simulink library "powerlib"  (Simulink 6.0)
settings: Solver=ode45  SolverMode=SingleTasking  StartTime=0.0  StopTime=10.0  RelTol=1e-3
undefined symbols (not defined in the file or in its folder): com, ctrl1, Da, DiscIntNeverNeededParam, dtha, etat, FA, find_system, Ha, j, Ka, Ki, Kv, q0, Rground, sel, st_a, st_b, st_c, sta, stb, stc, T1, T2, T3, T4
libraries: powerlib_models x30, powerlib x25, simulink_extras x6, powerlib_extras x3, simulink x2
(part 2 of 7)

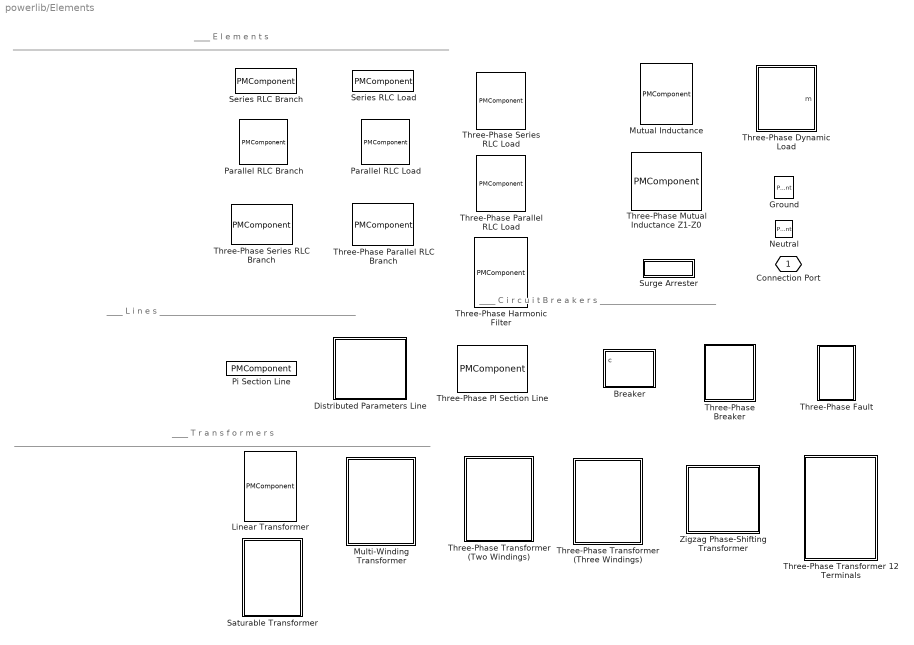
== system powerlib/Elements ==
  note: ____ T r a n s f o r m e r s ________________________________________________________________________________________________________
  note: ____ C i r c u i t B r e a k e r s _____________________________
  note: ____ L i n e s _________________________________________________
  note: ____ E l e m e n t s _____________________________________________________________________________________________________________
  Breaker : Subsystem  mask(Breaker){BreakerResistance=0.01, InitialState=0, SnubberResistance=1e6, SnubberCapacitance=inf, SwitchingTimes=[ 1/60  5/60 ], External=on, Measurements=None}
      mask prompts: BreakerResistance "Breaker resistance Ron (Ohm):"; InitialState "Initial state ( 0 for 'open' , 1 for 'closed' ):"; SnubberResistance "Snubber resistance Rs (Ohms):"; SnubberCapacitance "Snubber capacitance Cs (F):"; SwitchingTimes "Switching times (s):"; External "External control of switching times"
      mask help:
      | Implements a circuit breaker with internal resistance Ron. Ron is required by the
      | model  and cannot be set to zero.
      |
      | When the external control mode is selected, a Simulink  logical signal is used to
      | control the breaker operation.  When  the signal becomes greater than zero the
      | breaker closes instantaneously.  When it becomes zero, the breaker opens at the
      | next current zero-crossing.
      mask init:
      | block = gcb;
      | [p0,p1,p3,s1,s2,com,switchings]=powericon('Breaker',InitialState,SnubberResistance,SnubberCapacitance,SwitchingTimes,External);
      | powericon('BreakerCback',block);
      | powericon('psbloadfunction',block,'goto','Initialize');
      settings: CopyFcn=powericon('psbloadfunction',gcb,'goto','UpdateGotoTag');
      mask Help: web(psbhelp);
      mask StyleString: edit,edit,edit,edit,edit,checkbox,popup(None|Branch voltage|Branch current|Branch voltage and current)
      mask CallbackString: |||||powericon('BreakerCback',gcb);|
      mask Display: plot(p0,25,p1,75,[15,15,25,25,15],[55,45,45,55,55],[75,75,85,85,75],[55,45,45,55,55],[25,75],[50,p3],s1,s2)
  Distributed Parameters Line : Subsystem  mask(Distributed Parameters Line){Phases=3, Frequency=60, Resistance=[0.01273 0.3864], Inductance=[0.9337e-3  4.1264e-3], Capacitance=[12.74e-9 7.751e-9], Length=100, x1=[0 0 0 0; 0.0001244 0 0 0; 0.0002488 0 0 0; 0.0003733 0 0 0; 0.0004977 0 0 0; 0.0006221 0 0 0], x2=[0 0 0 0; 0.0001244 0 0 0; 0.0002488 0 0 0; 0.0003733 0 0 0; 0.0004977 0 0 0; 0.0006221 0 0 0], x3=[0 0 0 0; 0.0001244 0 0 0; 0.0002488 0 0 0; 0.0003733 0 0 0; 0.0004977 0 0 0; 0.0006221 0 0 0], x4=[0 0 0 0; 0.0001244 0 0 0; 0.0002488 0 0 0; 0.0003733 0 0 0; 0.0004977 0 0 0; 0.0006221 0 0 0], x5=0, Measurements=None}
      mask prompts: Phases "Number of phases N"; Frequency "Frequency used for R L C specification (Hz)"; Resistance "Resistance per unit length (Ohms/km)   [N*N matrix] or [R1 R0 R0m]"; Inductance "Inductance per unit length (H/km) [N*N matrix ] or [L1 L0 L0m]"; Capacitance "Capacitance per unit length (F/km) [N*N matrix] or [C1 C0 C0m]"; Length "Line length (km)"; x1 "v1 init"; x2 "v2 init"; x3 "I1 init"; x4 "I2 init"; x5 "time delay init"
      mask help:
      | Implements a N-phases distributed parameter line model. The R,L, and C line parameters are specified by [NxN] matrices.
      |
      | To model a two-, three-, or a six-phase symetrical line you can either specify complete [NxN] matrices or simply enter sequence parameters vectors: the  positive and zero sequence parameters for a two-phase or  three-phase transposed  line, plus the mutual zero-sequence for a  six-phase transposed  line  (2 coupled 3-phase lines).
      mask init:
      | Block = gcb;
      | powericon('DistributedParameterLineIcon',Block);
      | powericon('psbloadfunction',Block,'gotofrom','Initialize');
      | Ts = powericon('DistributedParameterLineInit',Block);
      | powericon('DistributedParameterLineCback',Block);
      settings: CopyFcn=powericon('psbloadfunction',gcb,'gotofrom','UpdateGotoTag');
      mask Help: web(psbhelp);
      mask StyleString: edit,edit,edit,edit,edit,edit,edit,edit,edit,edit,edit,popup(None|Phase-to-ground voltages)
      mask CallbackString: powericon('DistributedParameterLineCback',gcb);|||||||||||
      mask Display: plot([0 20 20 80 80 100 80 80 20 20],[0 0 5 5 0 0 0 -5 -5 0]+100,[0 20 20 80 80 100 80 80 20 20],[0 0 5 5 0 0 0 -5 -5 0]+60,[0 20 20 80 80 100 80 80 20 20],[0 0 5 5 0 0 0 -5 -5 0]+20,0,0,100,120)
  Ground : PMComponent  Orientation=down  PhysicalDomain=powersysdomain  LeftPortType=p1  RightPortType=p1  LConnTagsString=a
      settings: CopyFcn=set_param(gcb,'ShowName','off')
      mask Type: Ground
      mask Description: Ground connection.
      mask Help: web(psbhelp);
      mask Display: plot(-10,-10,10,10,-[5 5],[-10 10],[0 0],[-5 5],-[-5 -5],[-2.5 2.5],-[15 5],[0 0])
  Linear Transformer : PMComponent  PhysicalDomain=powersysdomain  LeftPortType=p1  RightPortType=p1  LConnTagsString=a|b  RConnTagsString=A|B|C|D  mask(Linear Transformer){NominalPower=[ 250e6 60 ], winding1=[ 424.35e3  0.002  0.08 ], winding2=[ 181.87e3  0.002  0.08 ], ThreeWindings=on, winding3=[ 60e3 0.005 0.02 ], RmLm=[ 500 500 ], Measurements=None}
      mask prompts: NominalPower "Nominal power and frequency [Pn(VA) fn(Hz)]:"; winding1 "Winding 1 parameters [V1(Vrms) R1(pu) L1(pu)]:"; winding2 "Winding 2 parameters [V2(Vrms) R2(pu) L2(pu)]:"; ThreeWindings "Three windings transformer"; winding3 "Winding 3 parameters [V3(Vrms) R3(pu) L3(pu)]:"; RmLm "Magnetization resistance and reactance [Rm(pu) Lm(pu)]:"
      mask help: Three windings linear transformer.
      mask init:
      | powericon('psbcallbacks',gcb,'Linear Transformer');
      mask Help: web(psbhelp);
      mask StyleString: edit,edit,edit,checkbox,edit,edit,popup(None|Winding voltages|Winding currents|Magnetization current|All voltages and currents)
      mask CallbackString: |||powericon('psbcallbacks',gcb,'Linear Transformer');|||
      mask Display:
      | plot(-85,-100,85,100,[-85 -45 -44 -34 -26 -21 -20 -22 -28 -37 -47 -57 -63 -63 -54 -44 -34 -26 -21 -20 -22 -28 -37 -47 -57 -63 -63 -54 -44 -34 -26 -21 -20 -22 -28 -37 -47 -57 -63 -63 -54 -44 -34 -26 -21 -20 -22 -28 -37 -45 -45 -85],[-50 -50 -50 -49 -45 -39 -33 -26 -21 -18 -17 -19 -22 -22 -26 -27 -25 -22 -16 -9 -3 2 6 6 4 1 1 -3 -4 -2 2 7 14 20 26 29 30 28 24 24 21 20 21 25 31 37 44 49 50 50 50 50],[85 45 44 34 26 21 20 22 28 37 47 57 63 63 54 44 34 26 21 20 22 28 37 47 57 63 63 54 44 34 26 21 20 22 28 37 47 57 63 63 54 44 34 26 21 20 22 28 37 45 45 85],[25 25 25 25.5 27.5 30.5 33.5 37 39.5 41 41.5 40.5 39 39 37 36.5 37.5 39 42 45.5 48.5 51 53 53 52 50.5 50.5 48.5 48 49 51 53.5 57 60 63 64.5 65 64 62 62 60.5 60 60.5 62.5 65.5 68.5 72 74.5 75 75 75 75],[85 45 44 34 26 21 20 22 28 37 47 57 63 63 54 44 34 26 21 20 22 28 37 47 57 63 63 54 44 34 26 21 20 22 28 37 47 57 63 63 54 44 34 26 21 20 22 28 37 45 45 85],[-25 -25 -25 -25.5 -27.5 -30.5 -33.5 -37 -39.5 -41 -41.5 -40.5 -39 -39 -37 -36.5 -37.5 -39 -42 -45.5 -48.5 -51 -53 -53 -52 -50.5 -50.5 -48.5 -48 -49 -51 -53.5 -57 -60 -63 -64.5 -65 -64 -62 -62 -60.5 -60 -60.5 -62.5 -65.5 -68.5 -72 -74.5 -75 -75 -75 -75],[-5 -5],[70 -70],[5 5],[70 -70])
      | text(-85,0, '1')
      | text(70,50, '2')
      | text(70,-50, '3')
  Multi-Winding Transformer : Subsystem  mask(Multi-Winding Transformer){LeftWindings=1, RightWindings=3, TappedWindings=no taps, NumberOfTaps=2, NominalPower=[75e3 60], NominalVoltages=[ 14400  120  120 120 ], WindingResistances=[ 0.005  0.005  0.005  0.005], WindingInductances=[ 0.02  0.02  0.02  0.02 ], SetSaturation=off, Rm=50, Lm=50, Saturation=[ 0,0 ; 0.0024,1.2 ; 1.0,1.52 ], Hysteresis=off, DataFile='hysteresis.mat', Measurements=None, InitialFlux=0, TransfoNumber=1}
      mask prompts: LeftWindings "Number of windings on left side"; RightWindings "Number of windings on right side"; TappedWindings "Tapped winding"; NumberOfTaps "----  Number of taps (equally spaced):"; NominalPower "Nominal power and frequency [Pn(VA) fn(Hz)]:"; NominalVoltages "Winding nominal voltages [U1 U2 ... Un] (Vrms):"; WindingResistances "Winding resistances [R1 R2 ... Rn] (pu):"; WindingInductances "Winding leakage inductances [L1 L2 ... Ln] (pu):"; SetSaturation "Saturable core"; Rm "Magnetization resistance  Rm (pu)"; Lm "Magnetization reactance Lm (pu)"; Saturation "Saturation characteristic (pu) [ i1 ,  phi1 ;  i2 , phi2 ; ... ]"; Hysteresis "Simulate hysteresis"; DataFile "----  Hysteresis Data Mat file"; InitialFlux "Initial Flux (internal use)"; TransfoNumber "Device number (internal use)"
      mask help:
      | Implements a transformer with multiple windings. The number of windings can be
      | specified for the left side and for the right side of the block.  Taps can be added
      | to the upper left winding or  to the upper right winding.
      mask init:
      | block = gcb;
      | [lx,ly,rx,ry,hlx,hly,hrx,hry] = powericon('NWindingsTransformerIcon');
      | %
      | powerbase = NominalPower(1);
      | wbase = 2*pi*NominalPower(2);
      | if TappedWindings>1
      | 	voltbase = NominalVoltages(1)/(NumberOfTaps+1);
      | else
      |     voltbase = NominalVoltages(1);
      | end
      | BaseCurrent = (powerbase/voltbase)*sqrt(2);
      | BaseFlux = (voltbase/wbase)*sqrt(2);
      | %
      | if SetSaturation
      | 	Saturation = [-Saturation(size(Saturation,1):-1:2,:) ; Saturation(2:size(Saturation,1),:)];
      |     SaturationCurrent = [Saturation(:,1)*BaseCurrent]';
      |     SaturationFlux = [Saturation(:,2)*BaseFlux]';
      | 	if Hysteresis
      |         InitialSlope = 1;
      | 	    [Tolerances,HT,UpperFlux,LowerFlux,Current] = powericon('inithysteresis',DataFile,BaseFlux,BaseCurrent);
      | 	    if HT.UnitsPopup == 2
      | 		    % The hysteresis characteristic is in S.I.
      | 		    % consequentely we do not need to convert the in/out signals
      | 		    % of the sfunction
      | 		    BaseCurrent = 1;
      | 		    BaseFlux = 1;
      | 	    end
      | 	end
      | end
      | %
      | %powericon('NWindingsTransformerCback',block,0);
      | Ts = powericon('NWindingsTransformerInit',block);
      mask Help: web(psbhelp);
      mask StyleString: edit,edit,popup(no taps|taps on upper left winding|taps on upper right winding),edit,edit,edit,edit,edit,checkbox,edit,edit,edit,checkbox,edit,popup(None|Winding voltages|Winding currents|Flux and excitation current ( Imag + IRm )|Flux and magnetization current ( Imag )|All measurements (V I Flux)),edit,edit
      mask CallbackString: powericon('NWindingsTransformerCback',gcb,0);|powericon('NWindingsTransformerCback',gcb,0);|powericon('NWindingsTransformerCback',gcb,1);|powericon('NWindingsTransformerCback',gcb,1);|||||powericon('NWindingsTransformerCback',gcb,0);||||powericon('NWindingsTransformerCback',gcb,0);||||
      mask Display:
      | plot(-300,-200,300,200,lx,ly,rx,ry)
      | 
      | plot([-10,-10],[-180,180])
      | plot([10,10],[-180,180])
      | 
      | color('white')
      | plot(hlx,hly,hrx,hry)
  Mutual Inductance : PMComponent  PhysicalDomain=powersysdomain  LeftPortType=p1  RightPortType=p1  LConnTagsString=a|b|c  RConnTagsString=A|B|C  mask(Mutual Inductance){SelfImpedance1=[1.1 1.1e-03], SelfImpedance2=[ 1.1 1.1e-03], ThreeWindings=on, SelfImpedance3=[ 1.1 1.1e-03], MutualImpedance=[1.0 1.0e-03], Measurements=None}
      mask prompts: SelfImpedance1 "Winding 1 self impedance [R1(Ohm) L1(H)]:"; SelfImpedance2 "Winding 2 self impedance [R2(Ohm) L2(H)]:"; ThreeWindings "Three windings Mutual Inductance"; SelfImpedance3 "Winding 3 self impedance [R3(Ohm) L3(H)]:"; MutualImpedance "Mutual impedance [Rm(Ohm) Lm(H)]:"
      mask help: Implements three inductances with mutual coupling.
      mask init:
      | powericon('psbcallbacks',gcb,'Mutual Inductance');
      | x = [-40 0 0 1 5 11 17 24 29 32 33 31 28 28 24 23 25 28 34 41 47 52 56 56 54 51 51 47 46 48 52 57 64 70 76 79 80 78 74 74 71 70 71 75 81 87 94 99 100 100 100 140];
      | y = [0 0 1 11 19 24 25 23 17 8 -2 -12 -18 -18 -9 1 11 19 24 25 23 17 8 -2 -12 -18 -18 -9 1 11 19 24 25 23 17 8 -2 -12 -18 -18 -9 1 11 19 24 25 23 17 8 0 0 0];
      | bx = [-50,50];
      | by = [0,0];
      settings: AttributesFormatString=\n
      mask Help: web(psbhelp);
      mask StyleString: edit,edit,checkbox,edit,edit,popup(None|Winding voltages|Winding currents|Winding voltages and currents)
      mask CallbackString: ||powericon('psbcallbacks',gcb,'Mutual Inductance');|||
      mask Display: plot(-90,-75,90,85,x-50,-y*0.8+58,x-50,y*0.8+5,x-50,y*0.8-49,bx,by+30,bx,by-20)
  Neutral : PMComponent  Orientation=down  PhysicalDomain=powersysdomain  LeftPortType=p1  RightPortType=p1  LConnTagsString=a  mask(Neutral){NodeNumber=10}
      mask prompts: NodeNumber "Node number:"
      mask help: Implements a neutral point with a labeled number
      mask init:
      | strno=sprintf('\n\n%d',NodeNumber);
      settings: AttributesFormatString=node %<NodeNumber>  CopyFcn=set_param(gcb,'ShowName','off')
      mask Help: web(psbhelp);
      mask Display: plot(-5,-5,5,5,-[10 5 5 -5 5 5],[0 0 -5 0 5 0.0])
  Parallel RLC Branch : PMComponent  PhysicalDomain=powersysdomain  LeftPortType=p1  RightPortType=p1  LConnTagsString=a  RConnTagsString=__new0  mask(Parallel RLC Branch){Resistance=1, Inductance=1e-3, Capacitance=1e-6, Measurements=None}
      mask prompts: Resistance "Resistance R (Ohms):"; Inductance "Inductance L (H):"; Capacitance "Capacitance C (F):"
      mask help: Implements a parallel RLC branch.
      mask init:
      | [s1,s2,s3,s4,r1,r2,l1,l2,c1,c2,c3,c4,x1,x2,x3,x4] = powericon('Parallel RLC Branch',Resistance,Inductance,Capacitance);
      settings: AttributesFormatString=\n
      mask Help: web(psbhelp);
      mask StyleString: edit,edit,edit,popup(None|Branch voltage|Branch current|Branch voltage and current)
      mask Display: plot(s1,s2,s3,s4,r1,r2,l1,l2,c1,c2,c3,c4,x1,x2,x3,x4)
  Parallel RLC Load : PMComponent  PhysicalDomain=powersysdomain  LeftPortType=p1  RightPortType=p1  LConnTagsString=a  RConnTagsString=__new0  mask(Parallel RLC Load){NominalVoltage=1000, NominalFrequency=60, ActivePower=10e3, InductivePower=100, CapacitivePower=100, Measurements=None}
      mask prompts: NominalVoltage "Nominal voltage Vn (Vrms):"; NominalFrequency "Nominal frequency fn (Hz):"; ActivePower "Active power P (W):"; InductivePower "Inductive reactive Power QL (positive var):"; CapacitivePower "Capacitive reactive power Qc (negative var):"
      mask help: Implements a parallel RLC load.
      mask init:
      | [s1,s2,s3,s4,r1,r2,l1,l2,c1,c2,c3,c4,x1,x2,x3,x4] = powericon('Parallel RLC Load',ActivePower,InductivePower,CapacitivePower);
      settings: AttributesFormatString=\n
      mask Help: web(psbhelp);
      mask StyleString: edit,edit,edit,edit,edit,popup(None|Branch voltage|Branch current|Branch voltage and current)
      mask Display: plot(s1,s2,s3,s4,r1,r2,l1,l2,c1,c2,c3,c4,x1,x2,x3,x4)
  Pi Section Line : PMComponent  PhysicalDomain=powersysdomain  LeftPortType=p1  RightPortType=p1  LConnTagsString=__new0  RConnTagsString=__new0  mask(Pi Section Line){Frequency=60, Resistance=0.2568, Inductance=2e-3, Capacitance=8.6e-9, Length=100, PiSections=1, Measurements=None}
      mask prompts: Frequency "Frequency used for R L C specification (Hz)"; Resistance "Resistance per unit length (Ohms/km):"; Inductance "Inductance per unit length (H/km):"; Capacitance "Capacitance per unit length (F/km):"; Length "Length (km):"; PiSections "Number of pi sections:"
      mask help: PI section transmission line.
      mask init:
      | [s1,s2,s3,s4,r1,r2,l1,l2,c1,c2,c3,c4] = powericon('Series RLC Branch',Resistance,Inductance,Capacitance);
      settings: AttributesFormatString=\n
      mask Help: web(psbhelp);
      mask StyleString: edit,edit,edit,edit,edit,edit,popup(None|Input and output voltages|Input and output currents|All voltages and currents)
      mask Display: plot(0,0,100,100,[45,45],[21,60],[54,41],[60,60],[50,49,49,49,49],[21,29,38,47,60])
  Saturable Transformer : Subsystem  mask(Saturable Transformer){NominalPower=[250e6 60], Winding1=[ 424.35e3  0.002  0.08 ], Winding2=[ 181.87e3  0.002  0.08 ], ThreeWindings=on, Winding3=[ 181.87e3  0.002  0.08 ], Saturation=[ 0,0 ; 0.0024,1.2 ; 1.0,1.52 ], CoreLoss=[500], Hysteresis=off, DataFile='hysteresis.mat', Measurements=None, InitialFlux=0, TransfoNumber=1}
      mask prompts: NominalPower "Nominal power and frequency [Pn(VA) fn(Hz)]:"; Winding1 "Winding 1 parameters [V1(Vrms) R1(pu) L1(pu)]:"; Winding2 "Winding 2 parameters [V2(Vrms) R2(pu) L2(pu)]:"; ThreeWindings "Three windings transformer"; Winding3 "Winding 3 parameters [V3(Vrms) R3(pu) L3(pu)]:"; Saturation "Saturation characteristic [i1(pu) phi1(pu); i2 phi2; ...]:"; CoreLoss "Core loss resistance and initial flux [Rm(pu) phi0(pu)] or [Rm(pu)] only:"; Hysteresis "Simulate hysteresis"; DataFile "Hysteresis Data Mat file"; InitialFlux "Initial Flux (internal use)"; TransfoNumber "Device number (internal use)"
      mask help: Three windings linear transformer.
      mask init:
      | block = gcb;
      | [p1,p2,p3,p4,p5,p6,p7,p8,mot,t1]=powericon('SaturableTransformerIcon',ThreeWindings);
      | %
      | powerbase = NominalPower(1);
      | wbase = 2*pi*NominalPower(2);
      | voltbase = Winding1(1);
      | BaseCurrent = (powerbase/voltbase)*sqrt(2);
      | BaseFlux = (voltbase/wbase)*sqrt(2);
      | Saturation = [-Saturation(size(Saturation,1):-1:2,:) ; Saturation(2:size(Saturation,1),:)];
      | SaturationCurrent = [Saturation(:,1)*BaseCurrent]';
      | SaturationFlux = [Saturation(:,2)*BaseFlux]'; 
      | if length(CoreLoss)==2
      |     InitialFlux = CoreLoss(2)*BaseFlux;
      | end
      | if Hysteresis
      |     InitialSlope = 1;
      | 	[sfun_InitialFlux,Tolerances,HT,UpperFlux,LowerFlux,Current] = powericon('inithysteresis',DataFile,BaseFlux,BaseCurrent,InitialFlux);
      | 	if HT.UnitsPopup == 2
      | 		% The hysteresis characteristic is in S.I.
      | 		% consequentely we do not need to convert the in/out signals
      | 		% of the sfunction
      | 		BaseCurrent = 1;
      | 		BaseFlux = 1;
      | 	end	
      | end
      | %
      | Ts = powericon('SaturableTransformerInit',block);
      | powericon('SaturableTransformerCback',block);
      | powericon('psbloadfunction',block,'gotogotofrom','Initialize');
      settings: CopyFcn=powericon('psbloadfunction',gcb,'gotogotofrom','UpdateGotoTag');
      mask Help: web(psbhelp)
      mask StyleString: edit,edit,edit,checkbox,edit,edit,edit,checkbox,edit,popup(None|Winding voltages|Winding currents|Flux and excitation current ( Imag + IRm )|Flux and magnetization current ( Imag )|All measurements (V I Flux)),edit,edit
      mask CallbackString: |||powericon('SaturableTransformerCback',gcb);||||powericon('SaturableTransformerCback',gcb);||||
      mask Display:
      | plot(-85,-100,85,100,p1,p2,p3,p4,p5,p6,p7,p8);
      | text(-85,0, '1');
      | text(70,t1, '2');
      | text(70,-50, mot);
  Series RLC Branch : PMComponent  PhysicalDomain=powersysdomain  LeftPortType=p1  RightPortType=p1  LConnTagsString=__new0  RConnTagsString=__new0  mask(Series RLC Branch){Resistance=1, Inductance=1e-3, Capacitance=1e-6, Measurements=None}
      mask prompts: Resistance "Resistance (Ohms):"; Inductance "Inductance (H):"; Capacitance "Capacitance (F):"
      mask help: Implements a series RLC branch.
      mask init:
      | [s1,s2,s3,s4,r1,r2,l1,l2,c1,c2,c3,c4] = powericon('Series RLC Branch',Resistance,Inductance,Capacitance);
      mask Help: web(psbhelp);
      mask StyleString: edit,edit,edit,popup(None|Branch voltage|Branch current|Branch voltage and current)
      mask Display: plot(s1,s2,s3,s4,r1,r2,l1,l2,c1,c2,c3,c4)
  Series RLC Load : PMComponent  PhysicalDomain=powersysdomain  LeftPortType=p1  RightPortType=p1  LConnTagsString=a  RConnTagsString=__new0  mask(Series RLC Load){NominalVoltage=1000, NominalFrequency=60, ActivePower=10e3, InductivePower=100, CapacitivePower=100, Measurements=None}
      mask prompts: NominalVoltage "Nominal voltage Vn (Vrms):"; NominalFrequency "Nominal frequency fn (Hz):"; ActivePower "Active power P (W):"; InductivePower "Inductive reactive power QL (positive var):"; CapacitivePower "Capacitive reactive power Qc (negative var):"
      mask help: Implements a series RLC load.
      mask init:
      | [s1,s2,s3,s4,r1,r2,l1,l2,c1,c2,c3,c4] = powericon('Series RLC Load',ActivePower,InductivePower,CapacitivePower);
      settings: AttributesFormatString=\n
      mask Help: web(psbhelp);
      mask StyleString: edit,edit,edit,edit,edit,popup(None|Branch voltage|Branch current|Branch voltage and current)
      mask Display: plot(s1,s2,s3,s4,r1,r2,l1,l2,c1,c2,c3,c4)
  Surge Arrester : Subsystem  mask(Surge Arrester){ProtectionVoltage=500e+03, Columns=2, ReferenceCurrent=500, Segment1=[.955 50], Segment2=[1.0 25], Segment3=[.9915 16.5], Measurements=None, MoreParameters=off, BreakLoop=off}
      mask prompts: ProtectionVoltage "Protection voltage  Vref(V):"; Columns "Number of columns:"; ReferenceCurrent "Reference current per column Iref(A):"; Segment1 "Segment 1 characteristics [ k1 alpha1 ]:"; Segment2 "Segment 2 characteristics [ k2 alpha2 ]:"; Segment3 "Segment 3 characteristics [ k3 alpha3 ]:"; MoreParameters "------------------- Show additional parameters -------------------"; BreakLoop "Break Algebraic loop in discrete model"
      mask help: Implements a metal-oxide surge arrester.
      mask init:
      | block = gcb;
      | powericon('psbloadfunction',block,'gotofrom','Initialize');
      | Ts = powericon('SurgeArresterInit',block,BreakLoop);
      settings: CopyFcn=powericon('psbloadfunction',gcb,'gotofrom','UpdateGotoTag');
      mask Help: web(psbhelp);
      mask StyleString: edit,edit,edit,edit,edit,edit,popup(None|Branch voltage|Branch current|Branch voltage and current),checkbox,checkbox
      mask CallbackString: |||||||powericon('SurgeArresterCback',gcb);|
      mask Display: plot(-100,-45,100,45,[-100 -35],[0 0],[100 35],[0 0],[-30 -30],[40 -40],[-20 -20],[40 -40],[-10 -10],[40 -40],[0 0],[40 -40],[10 10],[-40 40],[20 20],[-40 40],[30 30],[-40 40])
  Three-Phase Dynamic Load : Subsystem  mask(Three-Phase Dynamic Load){NominalVoltage=[ 500e3 60 ], ActiveReactivePowers=[50e6 25e6], PositiveSequence=[0.994 -11.8], ExternalControl=off, NpNq=[1.3 2], TimeConstants=[0  0  0  0], MinimumVoltage=0.7, LoadFlowParameters=[4,0,0,0,0]}
      mask prompts: NominalVoltage "Nominal L-L voltage and frequency  [Vn(Vrms) fn(Hz)]:"; ActiveReactivePowers "Active & reactive power at initial voltage [Po(W) Qo(var)]:"; PositiveSequence "Initial positive-sequence voltage Vo [Mag(pu) Phase (deg.)]:"; ExternalControl "External control of PQ"; NpNq "Parameters [ np  nq ]:"; TimeConstants "Time constants [Tp1 Tp2 Tq1 Tq2]  (s):"; MinimumVoltage "Minimum voltage Vmin (pu):"; LoadFlowParameters "Load Flow parameters"
      mask help:
      | Implements a three-phase, three-wire dynamic load. Active  power P and reactive
      |  power Q absorbed by the load vary as function of positive-sequence voltage V
      | according to following equations:
      |
      |   If V>Vmin, P and Q vary as follows:
      |        P=Po*(V/Vo)^np*(1+Tp1.s)/(1+Tp2.s)
      |        Q=Qo*(V/Vo)^nq*(1+Tq1.s)/(1+Tq2.s)
      |   if V<Vmin
      |      Same equations with np=nq=2 (constant impedance load)
      |
      | Check 'External control of PQ'  to control power from a vectorized Simulink
      | signal  [P Q] .
      mask init:
      | block = gcb;
      | Ts = powericon('ThreePhaseDynamicLoadInit',block);
      | powericon('ThreePhaseDynamicLoadCback',block);
      | powericon('psbloadfunction',block,'gotofrom','Initialize');
      | %
      | Vnom=NominalVoltage(1); 
      | fnom=NominalVoltage(2);
      | P0=ActiveReactivePowers(1);
      | Q0=ActiveReactivePowers(2);
      | Mag_V0=PositiveSequence(1); 
      | Pha_V0=PositiveSequence(2);
      | V0_d=Mag_V0*cos(Pha_V0*pi/180);
      | V0_q=Mag_V0*sin(Pha_V0*pi/180);
      | np=NpNq(1);
      | nq=NpNq(2);
      | Tp1=TimeConstants(1); 
      | Tp2=TimeConstants(2); 
      | Tq1=TimeConstants(3); 
      | Tq2=TimeConstants(4);
      | Vbase=Vnom/sqrt(3)*sqrt(2);
      | % initial value of positive-sequence current I1
      | I1_init=(P0-j*Q0)/((V0_d-j*V0_q)*Vnom)/sqrt(3)*sqrt(2);
      | Mag_ia=abs(I1_init);
      | Phase_ia=angle(I1_init)*180/pi;
      | %
      | Vmin=MinimumVoltage;
      | PQext=ExternalControl;
      | a=exp(j*2*pi/3);
      settings: CopyFcn=powericon('psbloadfunction',gcb,'gotofrom','UpdateGotoTag');
      mask Help: web(psbhelp)
      mask CallbackString: |||powericon('ThreePhaseDynamicLoadCback',gcb);||||
      mask Display:
      | plot(-45,-45,45,45,[0,9,18,24,29,30,29,24,18,9,0,-9,-18,-24,-29,-30,-29,-24,-18,-9,0]*.9,[30,29,24,18,9,0,-9,-18,-24,-29,-30,-29,-24,-18,-9,0,9,18,24,29,30]*.9)
      | plot([0,0,10,0,-10,0]*1.1,[15,-5,-5,-15,-5,-5]*1.1)
  Three-Phase Harmonic Filter : PMComponent  Orientation=down  PhysicalDomain=powersysdomain  LeftPortType=p1  RightPortType=p1  LConnTagsString=A|B|C  RConnTagsString=n  mask(Three-Phase Harmonic Filter){FilterType=Double-tuned, FilterConnection=Y (neutral), ParNom=[315e3 60], Qc=49e6, Fr=[5*60], Frd=[11*60 13*60], Q=16, Measurements=None}
      mask prompts: FilterType "Type of filter:"; FilterConnection "Filter connection:"; ParNom "Nominal L-L voltage and frequency  [Vn(Vrms) fn(Hz)]:"; Qc "Nominal reactive power (var):"; Fr "Tuning frequency (Hz)"; Frd "Tuning frequencies [ Fr1 (Hz)   Fr2 (Hz) ]"; Q "Quality factor (Q):"
      mask help:
      | Implements a three-phase harmonic filter.
      | The filter is built up from passive RLC components. Their values are computed using the specified  nominal reactive power, tuning frequency (ies) and quality factor.
      mask init:
      | % Data for drawing command (Icon)
      | cx0=[0 0];
      | a=-10.5;
      | cy0=[0 a];
      | cx1=[-8 8];
      | cy1=[0 0]+a;
      | cx2=[-8 8];
      | cy2=[-5 -5]+a;
      | cx3=[0 0];
      | cy3=[a-5 a-5-11.5];
      | %
      | lx0=[0 0];
      | a=-8;
      | ly0=[0 a];
      | lx1=[0 1.4 4.3 5.7 7.1 7.7 8 7.7 7.1 5.7 4.3 1.4 0];
      | ly1=[0 0 -0.3 -0.6 -1.2 -1.5 -2.25 -3 -3.3 -3.9 -4.2 -4.5 -4.5]+a;
      | lx2=lx1;
      | ly2=ly1-4.5;
      | lx3=lx1;
      | ly3=ly1-9;
      | lx4=[0 0];
      | ly4=[a-13.5 a-13.5-5.5];
      | %
      | rx0=[0 0];
      | a=-5;
      | ry0=[0 a];
      | rx1=[0 3.8 -3.8 3.8 -3.8 3.8 -3.8 0];
      | ry1=[0 -2.5 -5 -7.5 -10 -12.5 -15 -17.5]+a;
      | rx2=[0 0];
      | ry2=[a-17.5 a-17.5-4.5];
      | %
      | switch FilterType
      | case 1,   % Single-tuned
      | 	C1_xo=50; C1_yo=85;
      | 	L1_xo=50;L1_yo=64;
      | 	R1_xo=50;R1_yo=37;
      | 	C2_xo=C1_xo;C2_yo=C1_yo;
      | 	L2_xo=L1_xo;L2_yo=L1_yo;
      |     s1x=[C2_xo C2_xo];s2x=s1x;s1y=[C2_yo C2_yo];s2y=s1y;
      |     s3x=s1x;s4x=s3x;s3y=s1y;s4y=s2y;
      | case 2,   % Double-tuned
      | 	C2_xo=78; C2_yo=40;
      | 	L2_xo=22;L2_yo=40;
      | 	C1_xo=50; C1_yo=85;
      | 	L1_xo=50;L1_yo=66;
      | 	R1_xo=50;R1_yo=40;
      |     s1x=[L2_xo C2_xo];s2x=s1x;s1y=[40 40];s2y=[13 13];
      |     s3x=s1x;s4x=s3x;s3y=s1y;s4y=s2y;
      | case 3,   % High-pass
      | 	C1_xo=50; C1_yo=75;
      | 	L1_xo=33;L1_yo=48;
      | 	R1_xo=67;R1_yo=48;
      |     C2_xo=C1_xo;C2_yo=C1_yo;
      | 	L2_xo=L1_xo;L2_yo=L1_yo;
      |     s1x=[L1_xo R1_xo];s2x=s1x;s1y=[48 48];s2y=[21 21];
      |     s3x=[C1_xo C1_xo];s4x=s3x;s3y=[21 13];s4y=[85 C1_yo];
      | case 4,   % C-type High-pass
      | 	C2_xo=33; C2_yo=58;
      | 	C1_xo=50; C1_yo=85;
      | 	L1_xo=33;L1_yo=40;
      | 	R1_xo=67;R1_yo=51;
      |     L2_xo=L1_xo;L2_yo=L1_yo;
      |     s1x=[R1_xo C2_xo];s2x=s1x;s1y=[C2_yo C2_yo];s2y=[13 13];
      |     s3x=[R1_xo R1_xo];s4x=s3x;s3y=[R1_yo C2_yo];s4y=[13 25];
      | end
      | %
      | switch FilterConnection
      | case 1,   % Y (grounded)
      |     g_xo=50;g_yo=13;
      | 	gx1=[0 0];
      |     gy1=[0 -7];
      |     gx2=[-5.5 5.5];
      |     gy2=[-7 -7];
      |     gx3=[-3 3];
      |     gy3=gy2-2;
      |     gx4=[-1.5 1.5];
      |     gy4=gy2-4;
      | case 2,   % Y (floating)
      |     g_xo=50;g_yo=13;
      | 	gx1=[0 0];
      |     gy1=[0 -10];
      |     gx2=[-4 4];
      |     gy2=[-10 -10];
      |     gx3=[-4 -4];
      |     gy3=[-7 -10];
      |     gx4=[4 4];
      |     gy4=gy3;
      | case 3,   % Y (neutral)
      | 	g_xo=50;g_yo=13;
      | 	gx1=[0 0];
      |     gy1=[0 -11];
      |     gx2=gx1;
      |     gy2=gy1;
      |     gx3=gx1;
      |     gy3=gy1;
      |     gx4=gx1;
      |     gy4=gy1;
      | case 4,   % Delta
      | 	g_xo=50;g_yo=13;
      | 	gx1=[0 0];
      |     gy1=[0 -7];
      |     gx2=[8 14];
      |     gy2=[1 1]-10;
      |     gx3=[8 11];
      |     gy3=[1 6]-10;
      |     gx4=[11 14];
      |     gy4=[6 1]-10;
      | end
      settings: AttributesFormatString=\n
      mask Help: web(psbhelp);
      mask StyleString: popup(Single-tuned|Double-tuned|High-pass|C-type High-pass),popup(Y (grounded)|Y (floating)|Y (neutral)|Delta),edit,edit,edit,edit,edit,popup(None|Branch voltages|Branch currents|Branch voltages and currents)
      mask CallbackString: powericon('ThreePhaseHarmonicFilterCback',gcb);|powericon('ThreePhaseHarmonicFilterCback',gcb);||||||
      mask Display:
      | plot(12,0,88,95)
      | plot(C1_xo+cx0,C1_yo+cy0,C1_xo+cx1,C1_yo+cy1,C1_xo+cx2,C1_yo+cy2,C1_xo+cx3,C1_yo+cy3)
      | plot(L1_xo+lx0,L1_yo+ly0,L1_xo+lx1,L1_yo+ly1,L1_xo+lx2,L1_yo+ly2,L1_xo+lx3,L1_yo+ly3,L1_xo+lx4,L1_yo+ly4)
      | plot(R1_xo+rx0,R1_yo+ry0,R1_xo+rx1,R1_yo+ry1,R1_xo+rx2,R1_yo+ry2)
      | plot(C2_xo+cx0,C2_yo+cy0,C2_xo+cx1,C2_yo+cy1,C2_xo+cx2,C2_yo+cy2,C2_xo+cx3,C2_yo+cy3)
      | plot(L2_xo+lx0,L2_yo+ly0,L2_xo+lx1,L2_yo+ly1,L2_xo+lx2,L2_yo+ly2,L2_xo+lx3,L2_yo+ly3,L2_xo+lx4,L2_yo+ly4)
      | plot(s1x,s1y,s2x,s2y,s3x,s3y,s4x,s4y)
      | plot(g_xo+gx1,g_yo+gy1,g_xo+gx2,g_yo+gy2,g_xo+gx3,g_yo+gy3,g_xo+gx4,g_yo+gy4)
      | port_label('LConn', 1, 'A')
      | port_label('LConn', 2, 'B')
      | port_label('LConn', 3, 'C')
  Three-Phase Mutual Inductance Z1-Z0 : PMComponent  PhysicalDomain=powersysdomain  LeftPortType=p1  RightPortType=p1  LConnTagsString=a|b|c  RConnTagsString=A|B|C  mask(Three-Phase Mutual Inductance Z1-Z0){PositiveSequence=[ 2  50e-3], ZeroSequence=[4  100e-3]}
      mask prompts: PositiveSequence "Positive-sequence parameters : [R1 (Ohms) L1 (H)]"; ZeroSequence "Zero-sequence parameters :     [R0 (Ohms) L0 (H)]"
      mask help:
      | This block implements a three phase impedance with mutual
      | coupling between phases.  Self impedances and mutual
      | impedances are set by entering positive and zero sequences
      | parameters.
      mask init:
      | [s1,s2,s3,s4,lp1,lp2,ls1,ls2,lt1,lt2]=powericon('3-phase RL  positive & zero-sequence impedance',PositiveSequence,ZeroSequence);
      settings: AttributesFormatString=\n
      mask Help: web(psbhelp);
      mask Display:
      | plot(-85,-75,85,75,lp1,lp2,ls1,ls2,lt1,lt2);
      | port_label('RConn', 1, 'A')
      | port_label('RConn', 2, 'B')
      | port_label('RConn', 3, 'C')
      | port_label('LConn', 1, 'A')
      | port_label('LConn', 2, 'B')
      | port_label('LConn', 3, 'C')
  Three-Phase PI Section Line : PMComponent  PhysicalDomain=powersysdomain  LeftPortType=p1  RightPortType=p1  LConnTagsString=a|b|c  RConnTagsString=A|B|C  mask(Three-Phase PI Section Line){Frequency=60, Resistances=[ 0.01273 0.3864], Inductances=[ 0.9337e-3  4.1264e-3], Capacitances=[12.74e-9 7.751e-9], Length=100}
      mask prompts: Frequency "Frequency used for R L C specification (Hz) :"; Resistances "Positive- and zero-sequence resistances (Ohms/km)  [ R1  R0 ] :"; Inductances "Positive- and zero-sequence inductances (H/km) [ L1  L0 ] :"; Capacitances "Positive- and zero-sequence capacitances (F/km)  [ C1 C0 ] :"; Length "Line section length (km) :"
      mask help: This block implements a three-phase PI section line to represent a three-phase transmision line. This block represents only one PI section. To implements more that one PI section, you simply need to connect copies of this block in series.
      settings: AttributesFormatString=\n
      mask Help: web(psbhelp);
      mask Display:
      | plot(0,0,100,100,[20,20,80,80,90,80,80,20,20,10],[50,40,40,50,50,50,61,61,50,50],[56,39],[55,55],[44,44],[44,55],[53,50,50],[44,48,55])
      | port_label('RConn', 1, 'A')
      | port_label('RConn', 2, 'B')
      | port_label('RConn', 3, 'C')
      | port_label('LConn', 1, 'A')
      | port_label('LConn', 2, 'B')
      | port_label('LConn', 3, 'C')
  Three-Phase Parallel RLC Branch : PMComponent  PhysicalDomain=powersysdomain  LeftPortType=p1  RightPortType=p1  LConnTagsString=A|B|C  RConnTagsString=A|B|C  mask(Three-Phase Parallel RLC Branch){Resistance=1, Inductance=1e-3, Capacitance=1e-6, Measurements=None}
      mask prompts: Resistance "Resistance R (Ohms):"; Inductance "Inductance L (H):"; Capacitance "Capacitance C (F):"
      mask help: This block implements a three-phase parallel RLC branch.
      mask init:
      | [s1,s2,s3,s4,r1,r2,l1,l2,c1,c2,c3,c4,x1,x2,x3,x4] = powericon('Parallel RLC Branch',Resistance,Inductance,Capacitance);
      settings: AttributesFormatString=\n
      mask Help: See the help for the Parallel RLC Branch block.
      mask StyleString: edit,edit,edit,popup(None|Branch voltages|Branch currents|Branch voltages and currents)
      mask Display:
      | plot(s1-50,s2,s3+50,s4,r1,r2,l1,l2,c1,c2,c3,c4,x1,x2,x3,x4)
      | port_label('RConn', 1, 'A')
      | port_label('RConn', 2, 'B')
      | port_label('RConn', 3, 'C')
      | port_label('LConn', 1, 'A')
      | port_label('LConn', 2, 'B')
      | port_label('LConn', 3, 'C')
  Three-Phase Parallel RLC Load : PMComponent  Orientation=down  PhysicalDomain=powersysdomain  LeftPortType=p1  RightPortType=p1  LConnTagsString=A|B|C  mask(Three-Phase Parallel RLC Load){Configuration=Y (grounded), NominalVoltage=1000, NominalFrequency=60, ActivePower=10e3, InductivePower=100, CapacitivePower=100, Measurements=None}
      mask prompts: NominalVoltage "Nominal phase-to-phase voltage Vn (Vrms)"; NominalFrequency "Nominal frequency fn (Hz):"; ActivePower "Active power P (W):"; InductivePower "Inductive reactive Power QL (positive var):"; CapacitivePower "Capacitive reactive power Qc (negative var):"
      mask help: Implements a three-phase parallel RLC load.
      mask init:
      | [s1,s2,s3,s4,r1,r2,l1,l2,c1,c2,c3,c4,x1,x2,x3,x4] = powericon('Parallel RLC Load',ActivePower,InductivePower,CapacitivePower);
      | ground = Configuration==1;
      | neutral = Configuration==3;
      settings: AttributesFormatString=\n
      mask Help: web(psbhelp);
      mask StyleString: popup(Y (grounded)|Y (floating)|Y (neutral)|Delta),edit,edit,edit,edit,edit,popup(None|Branch voltages|Branch currents|Branch voltages and currents)
      mask CallbackString: powericon('psbcallbacks',gcb,'Three-Phase Parallel RLC Load');||||||
      mask Display:
      | plot(s1-50,s2,s3+30,s4,r1,r2,l1,l2,c1,c2,c3,c4,x1,x2,x3,x4)
      | 
      | plot( ground*[s3,s3],  ground*[-s2/4,s2/4])
      | plot( ground*[s3+10,s3+10], ground*[-s2/6,s2/6])
      | plot( ground*[s3+20,s3+20], ground*[-s2/10,s2/10])
      | 
      | plot( neutral*[ s3,s3+30], neutral*[0,0])
      | port_label('LConn', 1, 'A')
      | port_label('LConn', 2, 'B')
      | port_label('LConn', 3, 'C')
  Three-Phase Series RLC Branch : PMComponent  PhysicalDomain=powersysdomain  LeftPortType=p1  RightPortType=p1  LConnTagsString=A|B|C  RConnTagsString=A|B|C  mask(Three-Phase Series RLC Branch){Resistance=1, Inductance=1e-3, Capacitance=1e-6, Measurements=None}
      mask prompts: Resistance "Resistance R (Ohms):"; Inductance "Inductance L (H):"; Capacitance "Capacitance C (F):"
      mask help: This block implements a three-phase series RLC branch.
      mask init:
      | [s1,s2,s3,s4,r1,r2,l1,l2,c1,c2,c3,c4] = powericon('Series RLC Branch',Resistance,Inductance,Capacitance);
      settings: AttributesFormatString=\n
      mask Help: See the help for the Series RLC Branch Block.
      mask StyleString: edit,edit,edit,popup(None|Branch voltages|Branch currents|Branch voltages and currents)
      mask Display:
      | plot(s1-50,s2,s3+50,s4,r1,r2,l1,l2,c1,c2,c3,c4)
      | port_label('RConn', 1, 'A')
      | port_label('RConn', 2, 'B')
      | port_label('RConn', 3, 'C')
      | port_label('LConn', 1, 'A')
      | port_label('LConn', 2, 'B')
      | port_label('LConn', 3, 'C')
  Three-Phase Series RLC Load : PMComponent  Orientation=down  PhysicalDomain=powersysdomain  LeftPortType=p1  RightPortType=p1  LConnTagsString=A|B|C  mask(Three-Phase Series RLC Load){Configuration=Y (grounded), NominalVoltage=1000, NominalFrequency=60, ActivePower=10e3, InductivePower=100, CapacitivePower=100, Measurements=None}
      mask prompts: NominalVoltage "Nominal phase-to-phase voltage Vn (Vrms)"; NominalFrequency "Nominal frequency fn (Hz):"; ActivePower "Active power P (W):"; InductivePower "Inductive reactive power QL (positive var):"; CapacitivePower "Capacitive reactive power Qc (negative var):"
      mask help: Implements a series RLC load.
      mask init:
      | [s1,s2,s3,s4,r1,r2,l1,l2,c1,c2,c3,c4] = powericon('Series RLC Branch',ActivePower,InductivePower,CapacitivePower);
      | ground = Configuration==1;
      | neutral = Configuration==3;
      settings: AttributesFormatString=\n
      mask Help: web(psbhelp);
      mask StyleString: popup(Y (grounded)|Y (floating)|Y (neutral)|Delta),edit,edit,edit,edit,edit,popup(None|Branch voltages|Branch currents|Branch voltages and currents)
      mask CallbackString: powericon('psbcallbacks',gcb,'Three-Phase Series RLC Load');||||||
      mask Display:
      | plot(s1-60,s2,s3+80,s4,r1,r2,l1,l2,c1,c2,c3,c4)
      | 
      | plot( ground*[s3,s3], ground*[-s2/4,s2/4])
      | plot( ground*[s3+30,s3+30], ground*[-s2/6,s2/6])
      | plot( ground*[s3+60,s3+60], ground*[-s2/10,s2/10])
      | 
      | plot( neutral*[s3,s3+80], neutral*[0,0])
      | 
      | port_label('LConn', 1, 'A')
      | port_label('LConn', 2, 'B')
      | port_label('LConn', 3, 'C')
  Three-Phase Transformer (Three Windings) : Subsystem  mask(Three-Phase Transformer (Three Windings)){NominalPower=[ 250e6 , 60 ], Winding1Connection=Y, Winding1=[ 735e3 , 0.002 , 0.08 ], Winding2Connection=Y, Winding2=[ 315e3 , 0.002 , 0.08 ], Winding3Connection=Y, Winding3=[ 315e3 , 0.002 , 0.08 ], SetSaturation=off, Rm=500, Lm=500, Saturation=[ 0,0 ; 0.0024,1.2 ; 1.0,1.52 ], Hysteresis=off, DataFile='hysteresis', SetInitialFlux=off, InitialFluxes=[0.8 -0.8 0.7], Measurements=None, TransfoNumber=1}
      mask prompts: NominalPower "Nominal power and frequency  [ Pn(VA) , fn(Hz) ]"; Winding1Connection "Winding 1 (ABC) connection:"; Winding1 "Winding parameters [ V1 Ph-Ph(Vrms) , R1(pu) , L1(pu) ]"; Winding2Connection "Winding 2 (abc-2) connection:"; Winding2 "Winding parameters [ V2 Ph-Ph(Vrms) , R2(pu) , L2(pu) ]"; Winding3Connection "Winding 3 (abc-3) connection:"; Winding3 "Winding parameters [ V3 Ph-Ph(Vrms) , R3(pu) , L3(pu) ]"; SetSaturation "Saturable core"; Rm "Magnetization resistance  Rm(pu):"; Lm "Magnetization reactance Lm(pu)"; Saturation "Saturation characteristic (pu) [  i1 phi1;  i2 phi2 ; ...]"; Hysteresis "Simulate hysteresis"; DataFile "Hysteresis Data Mat file"; SetInitialFlux "Specify initial fluxes:"; InitialFluxes "[ phi0A phi0B phi0C] (pu)"; TransfoNumber "TransfoNumber (internal use only)"
      mask help: This block implements a three-phase transformer by using three single-phase transformers. Set the winding connection to 'Yn' when you want to access the neutral point of the Wye (for winding 1 and 3 only).
      mask init:
      | block = gcb;
      | [w1x,w1y,g1x,g1y,w2x,w2y,g2x,g2y,w3x,w3y,g3x,g3y,satx,saty,p]=powericon('ThreePhaseTransformer3Icon',Winding1Connection,Winding2Connection,Winding3Connection,SetSaturation);
      | %
      | [SaturationCurrent,SaturationFlux,InitialFlux1,InitialFlux2,InitialFlux3,BaseCurrent,BaseFlux] = powericon('ThreePhaseTransformerParam',block,NominalPower,Winding1Connection,Winding1,SetSaturation,Saturation,SetInitialFlux,InitialFluxes);
      | %
      | if SetSaturation & Hysteresis
      |     TransfoNumber1 = TransfoNumber;
      |     TransfoNumber2 = TransfoNumber+1;
      |     TransfoNumber3 = TransfoNumber+2;
      |     InitialSlope = 1;
      | 	[Tolerances,HT,UpperFlux,LowerFlux,Current] = powericon('inithysteresis',DataFile,BaseFlux,BaseCurrent);
      | end
      | %
      | powericon('psbcallbacks',block,'ThreeWindingsAccessToNeutrals',1);
      | powericon('psbcallbacks',block,'ThreeWindingsAccessToNeutrals',3);
      | Ts = powericon('ThreePhaseTransformer2Init',block);
      mask Help: web(psbhelp);
      mask StyleString: edit,popup(Y|Yn|Yg|Delta (D1)|Delta (D11)),edit,popup(Y|Yg|Delta (D1)|Delta (D11)),edit,popup(Y|Yn|Yg|Delta (D1)|Delta (D11)),edit,checkbox,edit,edit,edit,checkbox,edit,checkbox,edit,popup(None|Winding voltages|Winding currents|Fluxes and excitation currents ( Imag + IRm )|Fluxes and magnetization currents ( Imag )|All measurements (V I Fluxes)),edit
      mask CallbackString: |powericon('psbcallbacks',gcb,'ThreeWindingsAccessToNeutrals',1);||||powericon('psbcallbacks',gcb,'ThreeWindingsAccessToNeutrals',3);||powericon('psbcallbacks',gcb,'saturation3');||||powericon('psbcallbacks',gcb,'Hysteresis3');||powericon('psbcallbacks',gcb,'InitialFluxes3');|||
      mask Display:
      | plot(-180,-220,180,220,[-100,-40]*p,[0,0],[100,40]*p,[65,65],[100,40]*p,[-68,-68],
      | [-54 -38 -25 -17 -15 -19 -29 -43 -55 -54 -38 -25 -17 -15 -19 -29 -43 -55 -54 -38 -25 -17 -15 -19 -29 -43 -55 -54 -38 -25 -17 -15 -19 -29 -43 -55]*p,
      | [-98 -98 -92 -84 -74 -64 -56 -51 -50 -50 -48 -42 -34 -24 -14 -6 -1 0 0 3 8 17 27 36 44 49 50 50 53 58 67 77 86 94 99 99],
      | [54 38 25 17 15 19 29 43 55 54 38 25 17 15 19 29 43 55]*p,
      | [-117 -117 -111 -103 -93 -83 -75 -70 -69 -69 -67 -61 -53 -43 -33 -25 -20 -19],
      | [54 38 25 17 15 19 29 43 55 54 38 25 17 15 19 29 43 55]*p,
      | [13 16 21 30 40 49 57 62 63 63 66 71 80 90 99 107 112 112],
      | w1x*p,w1y,g1x,g1y,w2x*p,w2y,g2x,g2y,w3x*p,w3y,g3x,g3y,satx,saty)
  Three-Phase Transformer (Two Windings) : Subsystem  mask(Three-Phase Transformer (Two Windings)){NominalPower=[ 250e6 , 60 ], Winding1Connection=Y, Winding1=[ 735e3 , 0.002 , 0.08 ], Winding2Connection=Y, Winding2=[ 315e3 , 0.002 , 0.08 ], SetSaturation=off, Rm=500, Lm=500, Saturation=[ 0,0 ; 0.0024,1.2 ; 1.0,1.52 ], Hysteresis=off, DataFile='hysteresis', SetInitialFlux=off, InitialFluxes=[ 0.8 , -0.8 , 0.7 ], Measurements=None, TransfoNumber=1}
      mask prompts: NominalPower "Nominal power and frequency  [ Pn(VA) , fn(Hz) ]"; Winding1Connection "Winding 1 (ABC) connection :"; Winding1 "Winding parameters [ V1 Ph-Ph(Vrms) , R1(pu) , L1(pu) ]"; Winding2Connection "Winding 2 (abc) connection :"; Winding2 "Winding parameters [ V2 Ph-Ph(Vrms) , R2(pu) , L2(pu) ]"; SetSaturation "Saturable core"; Rm "Magnetization resistance  Rm (pu)"; Lm "Magnetization reactance Lm (pu)"; Saturation "Saturation characteristic (pu) [ i1 ,  phi1 ;  i2 , phi2 ; ... ]"; Hysteresis "Simulate hysteresis"; DataFile "Hysteresis Data Mat  file"; SetInitialFlux "Specify initial fluxes"; InitialFluxes "[ phi0A , phi0B , phi0C ] (pu):"; TransfoNumber "TransfoNumber (internal use only)"
      mask help: This block implements a three-phase transformer by using three single-phase transformers. Set the winding connection to 'Yn' when you want to access the neutral point of the Wye.
      mask init:
      | block = gcb;
      | [w1x,w1y,g1x,g1y,w2x,w2y,g2x,g2y,satx,saty]=powericon('ThreePhaseTransformer2Icon',Winding1Connection,Winding2Connection,SetSaturation);
      | %
      | [SaturationCurrent,SaturationFlux,InitialFlux1,InitialFlux2,InitialFlux3,BaseCurrent,BaseFlux] = powericon('ThreePhaseTransformerParam',block,NominalPower,Winding1Connection,Winding1,SetSaturation,Saturation,SetInitialFlux,InitialFluxes);
      | %
      | if SetSaturation & Hysteresis
      |     TransfoNumber1 = TransfoNumber;
      |     TransfoNumber2 = TransfoNumber+1;
      |     TransfoNumber3 = TransfoNumber+2;
      |     InitialSlope = 1;
      | 	[Tolerances,HT,UpperFlux,LowerFlux,Current] = powericon('inithysteresis',DataFile,BaseFlux,BaseCurrent);
      | end
      | %
      | powericon('psbcallbacks',block,'TwoWindingsAccessToNeutrals',1);
      | powericon('psbcallbacks',block,'TwoWindingsAccessToNeutrals',2);
      | Ts = powericon('ThreePhaseTransformer2Init',block);
      mask Help: web(psbhelp);
      mask StyleString: edit,popup(Y|Yn|Yg|Delta (D1)|Delta (D11)),edit,popup(Y|Yn|Yg|Delta (D1)|Delta (D11)),edit,checkbox,edit,edit,edit,checkbox,edit,checkbox,edit,popup(None|Winding voltages|Winding currents|Fluxes and excitation currents ( Imag + IRm )|Fluxes and magnetization currents ( Imag )|All measurements (V I Fluxes)),edit
      mask CallbackString: |powericon('psbcallbacks',gcb,'TwoWindingsAccessToNeutrals',1);||powericon('psbcallbacks',gcb,'TwoWindingsAccessToNeutrals',2);||powericon('psbcallbacks',gcb,'saturation2');||||powericon('psbcallbacks',gcb,'Hysteresis2');||powericon('psbcallbacks',gcb,'InitialFluxes2');|||
      mask Display:
      | plot(-180,-220,180,220,[-100,-40],[0,0],[100,40],[0,0],
      | [2 42 74 94 100 90 66 30 0 2 42 74 94 100 90 66 30 0 2 42 74 94 100 90 66 30 0 2 42 74 94 100 90 66 30 0]*.4-55,
      | [-45 -45 -34 -17 3 22 38 48 50 50 55 66 83 103 122 138 148 150 150 155 166 183 203 222 238 248 250 250 255 266 283 303 322 338 348 348]*0.5-75,
      | [2 42 74 94 100 90 66 30 0 2 42 74 94 100 90 66 30 0 2 42 74 94 100 90 66 30 0 2 42 74 94 100 90 66 30 0]*-.4+55,
      | [-45 -45 -34 -17 3 22 38 48 50 50 55 66 83 103 122 138 148 150 150 155 166 183 203 222 238 248 250 250 255 266 283 303 322 338 348 348]*0.5-75,
      | w1x,w1y,g1x,g1y,w2x,w2y,g2x,g2y,satx,saty)
  Three-Phase Breaker : Subsystem  LoadFcn=find_system(gcs,'FollowLinks', 'on', 'LookUnderMasks', 'all');  mask(Three-Phase Breaker){InitialState=open, SwitchA=on, SwitchB=on, SwitchC=on, SwitchTimes=[4/60  10/60], External=off, BreakerResistance=0.001, SnubberResistance=1e6, SnubberCapacitance=inf, Measurements=None}
      mask prompts: InitialState "Initial status of breakers"; SwitchA "Switching of phase A"; SwitchB "Switching of Phase B"; SwitchC "Switching of phase C"; SwitchTimes "Transition times (s)"; External "External control of switching times"; BreakerResistance "Breakers resistance Ron (ohms)"; SnubberResistance "Snubbers resistance Rp (Ohms)"; SnubberCapacitance "Snubbers capacitance Cp (Farad)"
      mask help:
      | Connect this block in series with the three-phase element
      | you want to switch. You can define the breaker timing directly
      | from the dialog box or apply an external logical signal. If you
      | check  the 'External control' box, the external control input
      | will appear.
      mask init:
      | [sta,stb,stc,etat,sw_times,switchings]=powericon('Three-Phase Breaker',InitialState,SwitchA,SwitchB,SwitchC,BreakerResistance,SwitchTimes,External);
      | if strcmp(InitialState,'open')
      |     p3=75;
      | else
      |     p3=50;
      | end
      | p0=-10;
      | p1=110;
      | 
      | if SnubberResistance==inf | SnubberCapacitance==0 | (SnubberResistance==inf & SnubberCapacitance==0)
      |     s1=0;
      |     s2=0;
      | else
      |     s1=[20,20,40,40,60,60,80,80,80,60,60,40,40];
      |     s2=[45,30,30,35,35,30,30,45,30,30,25,25,30];
      | end
      | powericon('ThreePhaseBreakerCback',gcb);
      mask Help: web(psbhelp)
      mask StyleString: popup(open|closed),checkbox,checkbox,checkbox,edit,checkbox,edit,edit,edit,popup(None|Breaker voltages|Breaker currents|Breaker voltages and currents)
      mask CallbackString: |||||powericon('ThreePhaseBreakerCback',gcb);||||
      mask Display: plot(p0,0,p1,100,[15,15,25,25,15],[55,45,45,55,55],[75,75,85,85,75],[55,45,45,55,55],[25,75],[50,p3],s1,s2)
  Three-Phase Fault : Subsystem  LoadFcn=find_system(gcs,'FollowLinks', 'on', 'LookUnderMasks', 'all');  mask(Three-Phase Fault){FaultA=on, FaultB=on, FaultC=on, FaultResistance=0.001, GroundFault=on, GroundResistance=0.001, External=off, SwitchStatus=[1 0], SwitchTimes=[ 1/60 5/60], InitialStates=[0 0 1], SnubberResistance=1e6, SnubberCapacitance=inf, Measurements=None}
      mask prompts: FaultA "Phase A Fault"; FaultB "Phase B Fault"; FaultC "Phase C Fault"; FaultResistance "Fault resistances  Ron (ohms) :"; GroundFault "Ground Fault"; GroundResistance "Ground resistance Rg (ohms) :"; External "External control of fault timing :"; SwitchStatus "Transition status [1,0,1 ...):"; SwitchTimes "Transition times (s):"; InitialStates "Initial status of fault [Phase A  Phase B  Phase C]:"; SnubberResistance "Snubbers resistance Rp (ohms) :"; SnubberCapacitance "Snubbers Capacitance Cp (Farad)"
      mask help:
      | Use this block to program a fault (short-circuit) between
      | any phase and the ground. You can define the fault timing
      | directly from the dialog box or apply an external logical signal.
      | If you check the 'External control' box , the external control
      | input will appear.
      mask init:
      | powerlibroot = which('powersysdomain');
      | powericon('ThreePhaseFaultCback',gcb);
      | PSBroot = powerlibroot(1:end-16);
      | %
      | [st_a,st_b,st_c,Rground,init_a,init_b,init_c,p7,p8,p9,p10,p11]=powericon('Three-Phase Fault',FaultResistance,GroundResistance,SwitchTimes,SwitchStatus,FaultA,FaultB,FaultC,GroundFault,InitialStates,External);
      | %
      mask Help: web(psbhelp)
      mask StyleString: checkbox,checkbox,checkbox,edit,checkbox,edit,checkbox,edit,edit,edit,edit,edit,popup(None|Fault voltages|Fault currents|Fault voltages and currents)
      mask CallbackString: ||||powericon('ThreePhaseFaultCback',gcb);||powericon('ThreePhaseFaultCback',gcb);||||||
      mask Display:
      | image(imread([PSBroot,'Fault.bmp'],'bmp'))
      | port_label('LConn', 1, 'A')
      | port_label('LConn', 2, 'B')
      | port_label('LConn', 3, 'C')
  Three-Phase Transformer 12 Terminals : Subsystem  LoadFcn=find_system(gcs,'FollowLinks', 'on', 'LookUnderMasks', 'all');  mask(Three-Phase Linear Transformer 12-Terminals){RatedPower=[ 10e6 60 ], Winding1=[ 10e3 0.002  0.05 ], Winding2=[ 25e3 0.002 0.05], RmXm=[ 200 200 ]}
      mask prompts: RatedPower "[Three-phase rated power(VA)  Frequency (Hz)]"; Winding1 "Winding 1 : [phase voltage(Vrms)  R(pu)  X(pu)] :"; Winding2 "Winding 2 : [phase voltage(Vrms)  R(pu)  X(pu)] :"; RmXm "Magnetizing branch : [Rm(pu)  Xm(pu)] :"
      mask help: This block implements three single-phase two-winding transformers . All winding terminals are accessible.
      mask init:
      | [p1,p2,p3,p4,p5,p6,p7,p8,p9,p10,p11,p12,p13,p14,p15,p16,p17,p18,p19,p20,p21,p22,p23,p24] = powericon('Three-phase Linear Transformer 12-terminals',RatedPower,Winding1,Winding2);
      | pnom=RatedPower(1)/3;
      | fnom=RatedPower(2);
      | u1=Winding1(1);
      | r1=Winding1(2);
      | x1=Winding1(3);
      | u2=Winding2(1);
      | r2=Winding2(2);
      | x2=Winding2(3);
      settings: AttributesFormatString=\n
      mask Display: plot(-130,-100,130,100,p1,p2,p3,p4,p13,p14,p15,p16,      p5,p6,p7,p8, p17,p18,p19,p20,     p9,p10,p11,p12,p21,p22,p23,p24  )
  Zigzag Phase-Shifting Transformer : Subsystem  mask(Zigzag Phase-Shifting Transformer){NominalPower=[ 100e6 60], PrimaryVoltage=10e3, SecondaryVoltage=[ 30e3  +15], SecondaryConnection=Y, Winding1=[ 0.002 0.08 ], Winding2=[ 0.002  0.08 ], Winding3=[ 0.002 0.08 ], SetSaturation=off, RmLm=[ 500 500 ], Rm=500, Saturation=[ 0,0 ; 0.0024,1.2 ; 1.0,1.52 ], Measurements=None, InitialFluxes=[0,0,0]}
      mask prompts: NominalPower "Nominal power and frequency [Pn(VA)  fn (Hz)] :"; PrimaryVoltage "Primary (zig-zag) nominal voltage Vp (VrmsPh-Ph) :"; SecondaryVoltage "Secondary nom. voltage & phase shift [V3(VrmsPh-Ph) Phi(Deg)]:"; SecondaryConnection "Secondary winding (abc) connection :"; Winding1 "Winding 1 (zig-zag) : [ R1(pu)  L1(pu)] :"; Winding2 "Winding 2 (zig-zag) : [ R2(pu)  L2(pu)] :"; Winding3 "Winding 3 (secondary) :  [ R3(pu)  L3(pu)] :"; SetSaturation "Saturable core"; RmLm "Magnetizing branch : [Rm(pu)  Lm(pu)] :"; Rm "Magnetization resistance  Rm (pu)"; Saturation "Saturation characteristic (pu) [ i1 ,  phi1 ;  i2 , phi2 ; ... ]"; InitialFluxes "Initial Fluxes"
      mask help: This block implements a three-phase phase-shifting transformer by using three single-phase three-winding transformers. Primary consists of windings 1 and 2 connected in zig-zag. All primary terminals are accessible. Secondary (winding 3) can be connected in wye or delta.
      mask init:
      | block = gcb;
      | [pzx1,pzy1,pzx2,pzy2,pzx3,pzy3,px1,py1,px2,py2,pgx1,pgy1,pgx2,pgy2,pgx3,pgy3,pgx4,pgy4,satx,saty]=powericon('ZigzagTransformerIcon',SecondaryVoltage,SecondaryConnection,SetSaturation);
      | %
      | alpha_deg = SecondaryVoltage(2);
      | if  alpha_deg==0,
      |    errordlg(' Phase shift cannot be zero' , 'Parameter error');
      | end
      | if  abs(alpha_deg)>=120,
      |    errordlg(' Phase shift cannot be larger than or equal to 120 degrees' , 'Parameter error');
      | end
      | powerbase = NominalPower(1)/3;
      | wbase = 2*pi*NominalPower(2);
      | voltbase = PrimaryVoltage/sqrt(3)*sin(2*pi/3-alpha_deg*pi/180)/sin(pi/3);
      | BaseCurrent = (powerbase/voltbase)*sqrt(2);
      | BaseFlux = (voltbase/wbase)*sqrt(2);
      | if SetSaturation==1
      |   Saturation = [-Saturation(size(Saturation,1):-1:2,:) ; Saturation(2:size(Saturation,1),:)];
      |   SaturationCurrent = [Saturation(:,1)*BaseCurrent]';
      |   SaturationFlux = [Saturation(:,2)*BaseFlux]'; 
      | end
      | InitialFlux1 = InitialFluxes(1)*BaseFlux;
      | InitialFlux2 = InitialFluxes(2)*BaseFlux;
      | InitialFlux3 = InitialFluxes(3)*BaseFlux;
      | 
      | powericon('ZigzagTransformerCback',block);
      | Ts = powericon('ZigzagTransformerInit',block);;
      mask Help: web(psbhelp)
      mask StyleString: edit,edit,edit,popup(Y|Yn|Yg|Delta D1(-30 deg.)|Delta D11(+30 deg.)),edit,edit,edit,checkbox,edit,edit,edit,popup(None|Phase voltages|Phase currents|Fluxes and excitation currents (Imag + IRm)|Fluxes and magnetization currents (Imag)|All measurements (V I Fluxes)),edit
      mask CallbackString: |||powericon('ZigzagTransformerCback',gcb);||||powericon('ZigzagTransformerCback',gcb);|||||
      mask Display:
      | plot(0,0,100,100,[19 31] ,[37 47], [49 37], [37 47], [34 34],[53 65]);
      | plot(0,0,100,100,pzx1,pzy1,pzx2,pzy2,pzx3,pzy3);
      | plot(0,0,100,100,px1,py1,px2,py2)
      | plot(0,0,100,100,pgx1,pgy1,pgx2,pgy2,pgx3,pgy3,pgx4,pgy4,satx,saty);
  Connection Port : PMIOPort  Tag=PMCPort  Port=1  Side=Left
